simulink model "test_big_model"  (R2021b)
settings: Solver=ode23tb  StartTime=0.0  StopTime=ctrl_tm  MaxStep=0.01  RelTol=1e-3
values from neighbouring files (symbols this model uses):
  A = J    (= 0.066829)    [test_big.m]    (also in test_small.m = 0.000254045)
  B = b_m + b + (b/(N^2*n_g))    (= 0.00010739)    [test_big.m]    (also in test_small.m = 6e-07)
  ctrl_k = k    (= 0)    [controller_init.m]    (also in controller_init2.m = 1; controller_init3.m = 1)
  ctrl_max_vel = max_vel    (= 6)    [controller_init.m]    (also in controller_init2.m = 10; controller_init3.m = 8)
  ctrl_mp = mp    (= 3)    [controller_init.m]    (also in controller_init2.m; controller_init3.m)
  ctrl_t1 = (tm-k*tm)/2    (= 3.75)    [controller_init.m]    (also in controller_init2.m = 0; controller_init3.m = 0)
  ctrl_t3 = ctrl_t1    (= 3.75)    [controller_init.m]    (also in controller_init2.m = 0; controller_init3.m = 0)
  ctrl_tm = tm    (= 7.5)    [controller_init.m]    (also in controller_init2.m = 3; controller_init3.m = 20)
  D = (mu_s*cos(angl) + sin(angl)) * r_p*(m_l+m_b)*g/(N*n_g)    [test_big.m]    (also in test_small.m = 0.113379075)
  Ke = 0.0537    [test_big.m]    (also in test_small.m = 0.0168)
  L = 0.0308e-3    (= 3.08e-05)    [test_big.m]    (also in test_small.m = 0.000333)
  max_i = 10    [test_big.m]
  MP_ON = 1    [test_big.m]
  N = (1:0.1:50)    [gear_ratio_code_1.m]    (also in test_big.m = 1; test_small.m = 1)
  R = 0.0821    [test_big.m]    (also in test_small.m = 3.17)
  r_p = 0.5e-1    (= 0.05)    [test_big.m]    (also in test_small.m = 0.005)
  USE_MAX_OP = 0    [test_big.m]
  V = 24    [test_big.m]    (also in test_small.m = 12)
undefined symbols (not defined in the file or in its folder): sigbuilder_block
libraries: slpidlib x1, simulink x1, eePwmGenerator x1
settings Model: Creator=marcelafunyah  LastModifiedBy=marcelafunyah

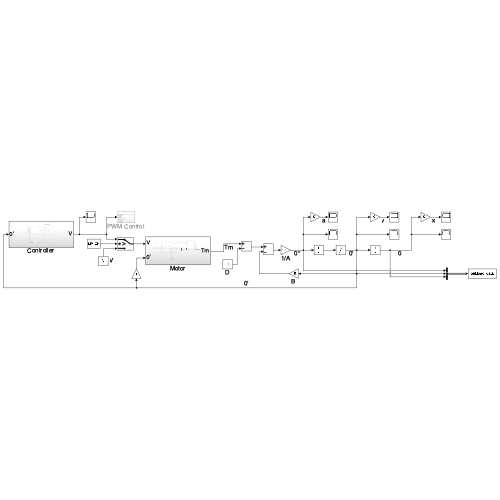
[thumbnail: Simulink's stored preview of the top-level diagram]
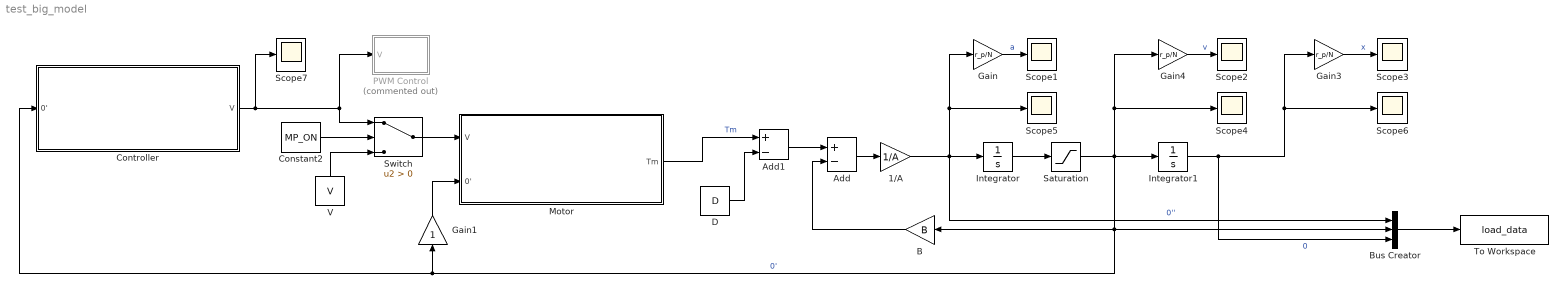
== system test_big_model ==
  1/A : Gain  Gain=1/A
  Add : Sum  Inputs=+-
  Add1 : Sum  Inputs=+-
  B : Gain  Gain=B
  Bus Creator : BusCreator  Inputs=3
  Constant2 : Constant  Value=MP_ON
  Controller : Subsystem
  D : Constant  Value=D
  Gain : Gain  Gain=r_p/N
  Gain1 : Gain
  Gain3 : Gain  Gain=r_p/N
  Gain4 : Gain  Gain=r_p/N
  Integrator : Integrator
  Integrator1 : Integrator
  Motor : Subsystem
  PWM Control : Subsystem  Commented=on
  Saturation : Saturate  UpperLimit=inf  LowerLimit=0
  Scope{1..7} (7 alike) : Scope
  Switch : Switch  Criteria=u2 > Threshold
  To Workspace : ToWorkspace  VariableName=load_data  SaveFormat=Timeseries  SampleTime=-1
  V : Constant  Value=V
  wires:
  Integrator/1 -> Saturation/1
  Integrator1/1 -> Bus Creator/3, Gain3/1, Scope6/1  "0"
  1/A/1 -> Bus Creator/1, Gain/1, Scope5/1, Integrator/1  "0''"
  B/1 -> Add/2
  Gain/1 -> Scope1/1  "a"
  Gain4/1 -> Scope2/1  "v"
  Gain3/1 -> Scope3/1  "x"
  Add/1 -> 1/A/1
  D/1 -> Add1/2
  Add1/1 -> Add/1
  Motor/1(Tm) -> Add1/1  "Tm"
  Controller/1(V) -> Scope7/1, PWM Control/1(V), Switch/1
  V/1 -> Switch/3
  Saturation/1 -> Gain4/1, Scope4/1, Controller/1(0'), Gain1/1, Bus Creator/2, B/1, Integrator1/1  "0'"
  Switch/1 -> Motor/1(V)
  Constant2/1 -> Switch/2
  Bus Creator/1 -> To Workspace/1
  Gain1/1 -> Motor/2(0')

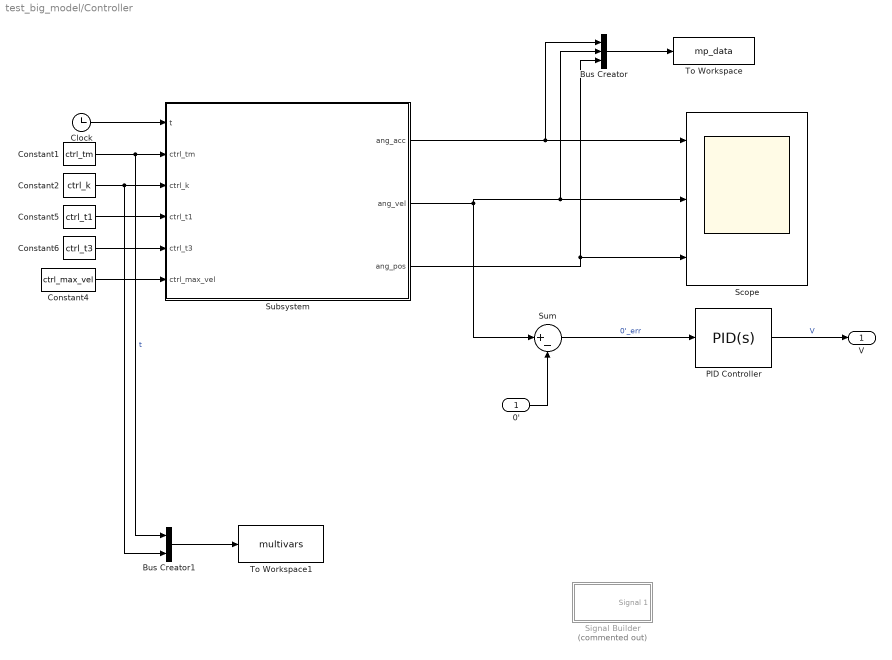
== system test_big_model/Controller ==
  0' : Inport
  Bus Creator : BusCreator  Inputs=3
  Bus Creator1 : BusCreator  Inputs=2
  Clock : Clock
  Constant1 : Constant  Value=ctrl_tm
  Constant2 : Constant  Value=ctrl_k
  Constant4 : Constant  Value=ctrl_max_vel
  Constant5 : Constant  Value=ctrl_t1
  Constant6 : Constant  Value=ctrl_t3
  PID Controller : slpidlib/PID Controller  Controller=PID  Form=Parallel  TimeDomain=Continuous-time  UseExternalTs=off  SampleTime=-1  IntegratorMethod=Forward Euler  FilterMethod=Forward Euler  ControllerParametersSource=internal  P=1452.99988960196  I=1492324.06717595  D=0.320852437052245  UseFilter=on  N=33719.8695903616  TunerSelectOption=Transfer Function Based (PID Tuner App)  InitialConditionSource=internal  InitialConditionForIntegrator=0  InitialConditionForFilter=0  DifferentiatorICPrevScaledInput=0  ExternalReset=none  TrackingMode=off  Kt=1  LimitOutput=on  SatLimitsSource=internal  UpperSaturationLimit=12  LowerSaturationLimit=0  LinearizeAsGain=on  AntiWindupMode=none  Kb=1  POutMin=[]  POutMax=[]  IOutMin=[]  IOutMax=[]  DOutMin=[]  DOutMax=[]  NOutMin=[]  NOutMax=[]  SumOutMin=[]  SumOutMax=[]  SaturationOutMin=[]  SaturationOutMax=[]  PParamMin=[]  PParamMax=[]  IParamMin=[]  IParamMax=[]  DParamMin=[]  DParamMax=[]  NParamMin=[]  NParamMax=[]  KbParamMin=[]  KbParamMax=[]  KtParamMin=[]  KtParamMax=[]  KbOutMin=[]  KbOutMax=[]  KtOutMin=[]  KtOutMax=[]  IntegratorOutMin=[]  IntegratorOutMax=[]  FilterOutMin=[]  FilterOutMax=[]  SumI1OutMin=[]  SumI1OutMax=[]  SumI2OutMin=[]  SumI2OutMax=[]  SumI3OutMin=[]  SumI3OutMax=[]  SumI4OutMin=[]  SumI4OutMax=[]  SumDOutMin=[]  SumDOutMax=[]  DifferentiatorOutMin=[]  DifferentiatorOutMax=[]  FilterDiffOutCoefMin=[]  FilterDiffOutCoefMax=[]  ReciprocalOutMin=[]  ReciprocalOutMax=[]  SumDenOutMin=[]  SumDenOutMax=[]  SumNumOutMin=[]  SumNumOutMax=[]  DivideOutMin=[]  DivideOutMax=[]  UdiffTsProdOutMin=[]  UdiffTsProdOutMax=[]  NTsProdOutMin=[]  NTsProdOutMax=[]  UintegralTsProdOutMin=[]  UintegralTsProdOutMax=[]  UngainTsProdOutMin=[]  UngainTsProdOutMax=[]  IntegratorContinuousStateAttributes=''  IntegratorStateMustResolveToSignalObject=off  IntegratorRTWStateStorageClass=Auto  FilterContinuousStateAttributes=''  FilterStateMustResolveToSignalObject=off  FilterRTWStateStorageClass=Auto  ParallelPVariant=InternalParameters  IdealPVariant=Disabled  IVariant=InternalParameters  DVariant=InternalParameters  IntegratorVariant=Continuous  SatVariant=Enabled  AWVariant=Passthrough  PCopyVariant=Disabled  TRVariant=Disabled  FdbkBlocksVariant=Forward  IdealPFdbkVariant=Disabled  SatFdbkVariant=Disabled  DerivativeFilterVariant=ContFilter  NVariant=InternalParameters  NCopyVariant=Disabled  FilterICVariant=InternalICsFilter  IntegratorICVariant=InternalICs  ExternalResetVariant=Disabled  TRSumVariant=Passthrough  SumFdbkVariant=Disabled  SumVariant=Sum_PID  TsampFilterVariant=InternalTs  TsampNgainVariant=Passthrough  TsampIntegralVariant=Passthrough  ExternalSaturationOutDataTypeStr=Inherit: Same as second input
  Scope : Scope  NumInputPorts=3
  Signal Builder : Subsystem  Tag=STV Subsys  Commented=on  LoadFcn=sigbuilder_block('load');  StartFcn=sigbuilder_block('start');  StopFcn=sigbuilder_block('stop');  ClipboardFcn=sigbuilder_block('clipboard');  mask(Sigbuilder block){tuvar=[0:10]}
      mask help: Simulink:masks:SigbuilderBlock_MD
      mask init:
      | if ~strcmp(get_param(bdroot(gcbh),'SimulationStatus'),'stopped') tuvar = sigbuilder_block('maskInit'); end
      settings: CopyFcn=sigbuilder_block('copy');  DeleteFcn=sigbuilder_block('delete');  ModelCloseFcn=sigbuilder_block('modelClose');  PreSaveFcn=sigbuilder_block('preSave');  PauseFcn=sigbuilder_block('pause');  ContinueFcn=sigbuilder_block('continue');  NameChangeFcn=sigbuilder_block('namechange');  OpenFcn=sigbuilder_block('open',[437.6 199.2 550.4 400 ]);  CloseFcn=sigbuilder_block('close');
      mask Display: plot(0, 0, 100, 100,[2, 2, 32, 32, 2], [68, 8, 8, 68, 68],[32, 2], [38, 38], [32, 19, 2],[53, 60, 44], [32, 17, 17, 2],[16, 16, 31, 31]);txt = getActiveGroup(gcbh);text(2, 100, txt,'verticalAlignment', 'top');
  Subsystem : Subsystem
  Sum : Sum  Inputs=|+-
  To Workspace : ToWorkspace  VariableName=mp_data  SaveFormat=Timeseries  SampleTime=-1
      settings: Save2DSignal=2-D array (concatenate along first dimension)
  To Workspace1 : ToWorkspace  VariableName=multivars  SaveFormat=Timeseries  SampleTime=-1
      settings: Save2DSignal=2-D array (concatenate along first dimension)
  V : Outport
  wires:
  Sum/1 -> PID Controller/1  "0'_err"
  PID Controller/1 -> V/1  "V"
  0'/1 -> Sum/2
  Bus Creator/1 -> To Workspace/1
  Subsystem/2(ang_vel) -> Bus Creator/2, Scope/2, Sum/1
  Subsystem/1(ang_acc) -> Bus Creator/1, Scope/1
  Subsystem/3(ang_pos) -> Bus Creator/3, Scope/3
  Clock/1 -> Subsystem/1(t)
  Constant1/1 -> Bus Creator1/1, Subsystem/2(ctrl_tm)  "t"
  Constant2/1 -> Bus Creator1/2, Subsystem/3(ctrl_k)
  Constant4/1 -> Subsystem/6(ctrl_max_vel)
  Bus Creator1/1 -> To Workspace1/1
  Constant6/1 -> Subsystem/5(ctrl_t3)
  Constant5/1 -> Subsystem/4(ctrl_t1)

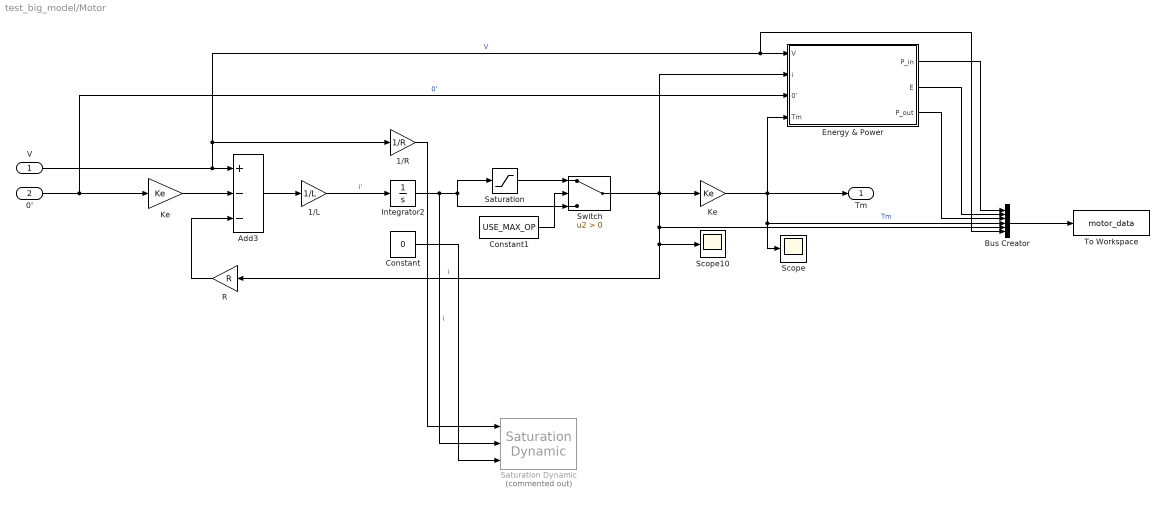
== system test_big_model/Motor ==
  V : Inport
  0' : Inport  Port=2
  1/L : Gain  Gain=1/L
  1/R : Gain  Gain=1/R
  Add3 : Sum  Inputs=+--
  Bus Creator : BusCreator  Inputs=6
  Constant : Constant  Value=0
  Constant1 : Constant  Value=USE_MAX_OP
  Energy & Power : Subsystem
  Integrator2 : Integrator
  Ke : Gain  Gain=Ke
  "Ke " : Gain  Gain=Ke
  R : Gain  Gain=R
  Saturation : Saturate  UpperLimit=max_i  LowerLimit=-inf
  Saturation Dynamic : simulink/Discontinuities/Saturation Dynamic  Commented=on  OutMin=[]  OutMax=[]  OutDataTypeStr=Inherit: Same as second input  OutDataType=fixdt(1, 16)  OutScaling=2^-10  DoSatur=off
  Scope : Scope
  Scope10 : Scope
  Switch : Switch  Criteria=u2 > Threshold
  To Workspace : ToWorkspace  VariableName=motor_data  SaveFormat=Timeseries  SampleTime=-1
  Tm : Outport
  wires:
  R/1 -> Add3/3
  Add3/1 -> 1/L/1
  "Ke "/1 -> Tm/1, Energy & Power/4(Tm), Scope/1, Bus Creator/4  "Tm"
  1/L/1 -> Integrator2/1  "i'"
  Ke/1 -> Add3/2
  V/1 -> Bus Creator/6, Energy & Power/1(V), 1/R/1, Add3/1  "V"
  0'/1 -> Ke/1, Energy & Power/3(0')  "0'"
  Integrator2/1 -> Switch/3, Saturation/1, Saturation Dynamic/2  "i"
  1/R/1 -> Saturation Dynamic/1
  Constant/1 -> Saturation Dynamic/3
  Bus Creator/1 -> To Workspace/1
  Energy & Power/3(P_out) -> Bus Creator/3
  Energy & Power/2(E) -> Bus Creator/2
  Energy & Power/1(P_in) -> Bus Creator/1
  Switch/1 -> Energy & Power/2(i), R/1, Scope10/1, Bus Creator/5, "Ke "/1  "i"
  Saturation/1 -> Switch/1
  Constant1/1 -> Switch/2

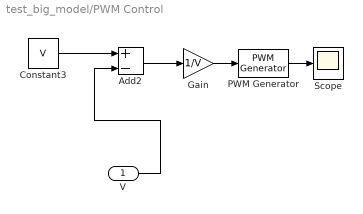
== system test_big_model/PWM Control ==
  V : Inport
  Add2 : Sum  Inputs=+-
  Constant3 : Constant  Value=V
  Gain : Gain  Gain=1/V
  PWM Generator : eePwmGenerator/PWM Generator  CarrCount=Up  Tper=0.001  Tdelay=0  Ts=0
  Scope : Scope
  wires:
  PWM Generator/1 -> Scope/1
  Gain/1 -> PWM Generator/1
  Constant3/1 -> Add2/1
  V/1 -> Add2/2
  Add2/1 -> Gain/1

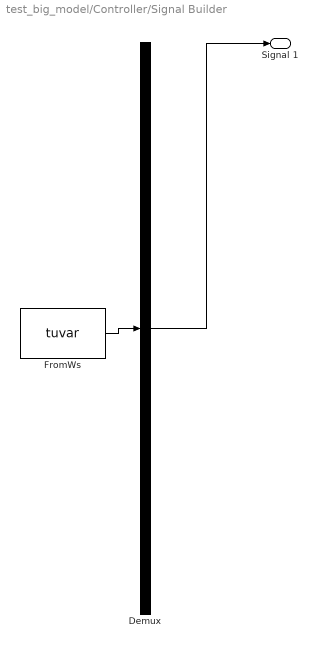
== system test_big_model/Controller/Signal Builder ==
  Demux : Demux  Tag=STV Demux  Outputs=1
      settings: DisplayOption=none
  FromWs : FromWorkspace  Tag=STV FromWs  VariableName=tuvar
      SigBuilderData=|
      | common.afterFinalStr = 'Extrapolate'
      | common.sampleTime = 0
      | dataSet.timeRange = [0 5]
      | dataSet.name = 'Group 1'
      | sbobj.Groups.Name = 'Group 1'
      | sbobj.Groups.Signals.Name = 'Signal 1'
      | sbobj.Groups.Signals.XData = [0 5]
      | sbobj.Groups.Signals.YData = [0.75 0.75]
      | sbobj.Groups.TimeRange = [0 5]
  Signal 1 : Outport  Tag=STV Outport
  wires:
  Demux/1 -> Signal 1/1
  FromWs/1 -> Demux/1

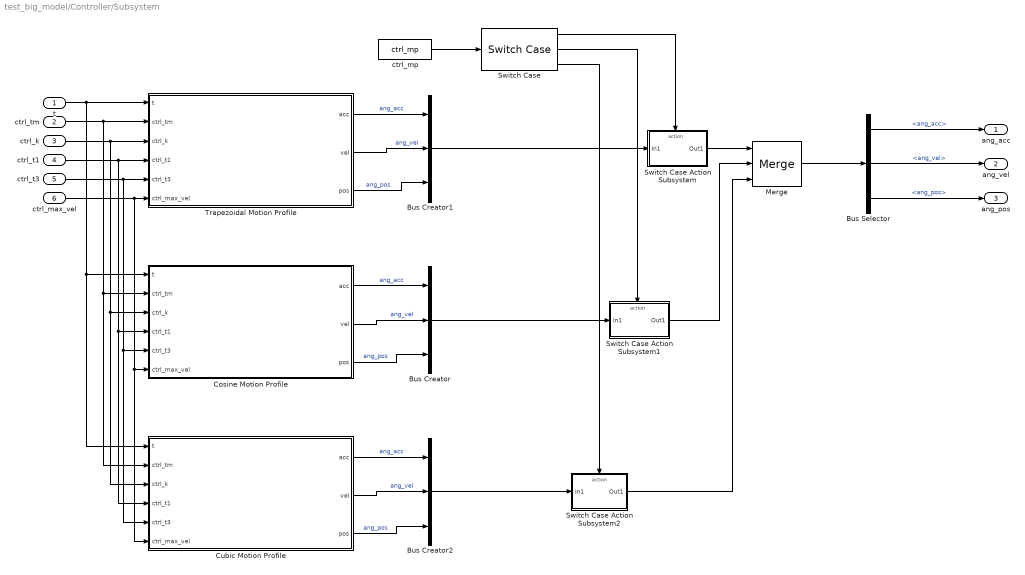
== system test_big_model/Controller/Subsystem ==
  t : Inport
  ctrl_tm : Inport  Port=2
  ctrl_k : Inport  Port=3
  ctrl_t1 : Inport  Port=4
  ctrl_t3 : Inport  Port=5
  ctrl_max_vel : Inport  Port=6
  Bus Creator : BusCreator  Inputs=3
  Bus Creator1 : BusCreator  Inputs=3
  Bus Creator2 : BusCreator  Inputs=3
  Bus Selector : BusSelector  OutputSignals=ang_acc,ang_vel,ang_pos
  Cosine Motion Profile : MATLAB Function  TreatAsAtomicUnit=on
  Cubic Motion Profile : MATLAB Function  TreatAsAtomicUnit=on
  Merge : Merge  Inputs=3
  Switch Case : SwitchCase  CaseConditions={1,2,3}  ShowDefaultCase=off
  Switch Case Action Subsystem : Subsystem  TreatAsAtomicUnit=on
  Switch Case Action Subsystem1 : Subsystem  TreatAsAtomicUnit=on
  Switch Case Action Subsystem2 : Subsystem  TreatAsAtomicUnit=on
  Trapezoidal Motion Profile : MATLAB Function  TreatAsAtomicUnit=on
  ctrl_mp : Constant  Value=ctrl_mp
  ang_acc : Outport
  ang_vel : Outport  Port=2
  ang_pos : Outport  Port=3
  wires:
  Cosine Motion Profile/1(acc) -> Bus Creator/1  "ang_acc"
  Cosine Motion Profile/3(pos) -> Bus Creator/3  "ang_pos"
  Cosine Motion Profile/2(vel) -> Bus Creator/2  "ang_vel"
  Switch Case/1 -> Switch Case Action Subsystem/Action
  Trapezoidal Motion Profile/1(acc) -> Bus Creator1/1  "ang_acc"
  Trapezoidal Motion Profile/2(vel) -> Bus Creator1/2  "ang_vel"
  Trapezoidal Motion Profile/3(pos) -> Bus Creator1/3  "ang_pos"
  Bus Creator1/1 -> Switch Case Action Subsystem/1(In1)
  Switch Case Action Subsystem/1(Out1) -> Merge/1
  Switch Case/2 -> Switch Case Action Subsystem1/Action
  Bus Creator/1 -> Switch Case Action Subsystem1/1(In1)
  Switch Case Action Subsystem1/1(Out1) -> Merge/2
  Merge/1 -> Bus Selector/1
  Bus Selector/1 -> ang_acc/1  "<ang_acc>"
  Bus Selector/2 -> ang_vel/1  "<ang_vel>"
  Bus Selector/3 -> ang_pos/1  "<ang_pos>"
  ctrl_mp/1 -> Switch Case/1
  Cubic Motion Profile/1(acc) -> Bus Creator2/1  "ang_acc"
  t/1 -> Cubic Motion Profile/1(t), Cosine Motion Profile/1(t), Trapezoidal Motion Profile/1(t)
  ctrl_max_vel/1 -> Cubic Motion Profile/6(ctrl_max_vel), Cosine Motion Profile/6(ctrl_max_vel), Trapezoidal Motion Profile/6(ctrl_max_vel)
  ctrl_tm/1 -> Cubic Motion Profile/2(ctrl_tm), Cosine Motion Profile/2(ctrl_tm), Trapezoidal Motion Profile/2(ctrl_tm)
  Cubic Motion Profile/2(vel) -> Bus Creator2/2  "ang_vel"
  ctrl_k/1 -> Cubic Motion Profile/3(ctrl_k), Cosine Motion Profile/3(ctrl_k), Trapezoidal Motion Profile/3(ctrl_k)
  Bus Creator2/1 -> Switch Case Action Subsystem2/1(In1)
  Cubic Motion Profile/3(pos) -> Bus Creator2/3  "ang_pos"
  Switch Case/3 -> Switch Case Action Subsystem2/Action
  Switch Case Action Subsystem2/1(Out1) -> Merge/3
  ctrl_t1/1 -> Cubic Motion Profile/4(ctrl_t1), Cosine Motion Profile/4(ctrl_t1), Trapezoidal Motion Profile/4(ctrl_t1)
  ctrl_t3/1 -> Cubic Motion Profile/5(ctrl_t3), Cosine Motion Profile/5(ctrl_t3), Trapezoidal Motion Profile/5(ctrl_t3)

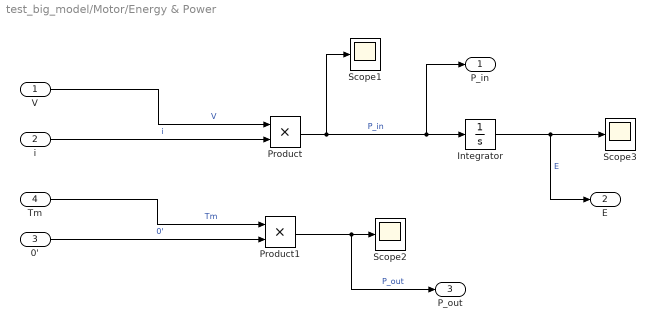
== system test_big_model/Motor/Energy & Power ==
  V : Inport
  i : Inport  Port=2
  0' : Inport  Port=3
  Tm : Inport  Port=4
  Integrator : Integrator
  Product : Product
  Product1 : Product
  Scope1 : Scope
  Scope2 : Scope
  Scope3 : Scope
  P_in : Outport
  E : Outport  Port=2
  P_out : Outport  Port=3
  wires:
  V/1 -> Product/1  "V"
  i/1 -> Product/2  "i"
  Product/1 -> P_in/1, Integrator/1, Scope1/1  "P_in"
  Integrator/1 -> E/1, Scope3/1  "E"
  Tm/1 -> Product1/1  "Tm"
  0'/1 -> Product1/2  "0'"
  Product1/1 -> P_out/1, Scope2/1  "P_out"

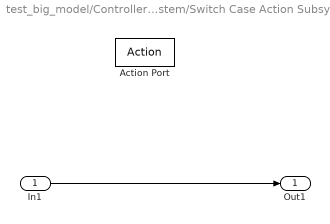
== system test_big_model/Controller/Subsystem/Switch Case Action Subsystem ==
  In1 : Inport
  Action Port : ActionPort  ActionPortLabel=case [ 1 ]:
  Out1 : Outport
  wires:
  In1/1 -> Out1/1

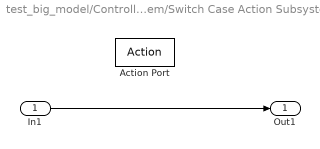
== system test_big_model/Controller/Subsystem/Switch Case Action Subsystem1 ==
  In1 : Inport
  Action Port : ActionPort  ActionPortLabel=case [ 2 ]:
  Out1 : Outport
  wires:
  In1/1 -> Out1/1

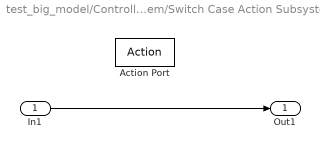
== system test_big_model/Controller/Subsystem/Switch Case Action Subsystem2 ==
  In1 : Inport
  Action Port : ActionPort  ActionPortLabel=case [ 3 ]:
  Out1 : Outport
  wires:
  In1/1 -> Out1/1

== matlab function test_big_model/Controller/Subsystem/Cosine Motion Profile ==
  data: t input; acc output; vel output; pos output; ctrl_tm input; ctrl_k input; ctrl_t1 input; ctrl_t3 input; ctrl_max_vel input
function [acc,vel,pos] = fcn(t, ctrl_tm, ctrl_k, ctrl_t1, ctrl_t3, ctrl_max_vel)

tm = ctrl_tm;
k = ctrl_k;

t1 = ctrl_t1;
t3 = ctrl_t3;

max_ang_vel = ctrl_max_vel;


% ta = 0;
% tb = ta + 0.5 * (tm - k*tm);
% tc = tb + k*tm;
% td = tm;
% 
% t_acc = tb - ta;
% t_dec = td - tc;


ta = 0;
tb = ta + t1;
tc = tb + k*tm;
td = tm;

t_acc = t1;
t_dec = t3;

thet1 = pi/t_acc;
thet3 = pi/t_dec;


if (t>=ta) && (t<=tb)
    ang_acc = max_ang_vel*(thet1*sin(thet1*t))/2;
    ang_vel = max_ang_vel*(1-cos(thet1*t))/2;
    ang_pos = max_ang_vel*(t-sin(thet1*t)/thet1)/2;

elseif (t>tb) && (t<=tc)
    ang_acc = 0;
    ang_vel = max_ang_vel;
    ang_pos = max_ang_vel*(t-t_acc/2);

elseif (t>tc) && (t<=td)
    tprm = t - tm + t_dec;
    ang_acc = -max_ang_vel*(thet3*sin(thet3*tprm))/2;
    ang_vel = max_ang_vel*(1+cos(thet3*tprm))/2;
    ang_pos = max_ang_vel*(tm - t_acc/2 - t_dec) + max_ang_vel*(tprm+sin(thet3*tprm)/thet3)/2;
else
    tprm = tm - tm + t_dec;
    ang_acc = 0;
    ang_vel = 0;
    ang_pos = max_ang_vel*(tm - t_acc/2 - t_dec) + max_ang_vel*(tprm+sin(thet3*tprm)/thet3)/2;
end



acc = ang_acc;
vel = ang_vel;
pos = ang_pos;

== matlab function test_big_model/Controller/Subsystem/Trapezoidal Motion Profile ==
  data: t input; acc output; vel output; pos output; ctrl_tm input; ctrl_k input; ctrl_t1 input; ctrl_t3 input; ctrl_max_vel input
function [acc,vel,pos] = fcn(t, ctrl_tm, ctrl_k, ctrl_t1, ctrl_t3, ctrl_max_vel)

    tm = ctrl_tm;
    k = ctrl_k;

    t1 = ctrl_t1;
    t3 = ctrl_t3;

    vel = ctrl_max_vel;

    ta = 0;
    tb = ta + t1;
    tc = tb + k*tm;
    td = tm;

    A1 =vel / t1;
    A2 =vel / t3;


    if (t>=ta) && (t<=tb)
        ang_acc = A1;
        ang_vel = A1 * t;
        ang_pos = 0.5 * A1 * t^2; 
    elseif (t>tb) && (t<=tc)
        ang_acc = 0;
        ang_vel = A1 * tb;
        ang_pos = (0.5 * A1 * tb^2) + (A1 * tb) * (t - tb); 
    elseif (t>tc) && (t<=td)
        ang_acc = -A2;
        ang_vel = (A1 * tb) - A2*(t-tc);
        ang_pos = (0.5 * A1 * tb^2) + (A1 * tb) * (tc - tb) + (A1 * tb) * (t - tc) + (A2 * tc) * (t - tc) - 0.5 * A2 * (t^2 - tc^2);
    else
        ang_acc = 0;
        ang_vel = 0;
        ang_pos = (0.5 * A1 * tb^2) + (A1 * tb) * (tc - tb) + (A1 * tb) * (tm - tc) + (A2 * tc) * (tm - tc) - 0.5 * A2 * (tm^2 - tc^2);
    end


acc = ang_acc;
vel = ang_vel;
pos = ang_pos;

== matlab function test_big_model/Controller/Subsystem/Cubic Motion Profile ==
  data: t input; acc output; vel output; pos output; ctrl_tm input; ctrl_k input; ctrl_t1 input; ctrl_t3 input; ctrl_max_vel input
function [acc,vel,pos] = fcn(t, ctrl_tm, ctrl_k, ctrl_t1, ctrl_t3, ctrl_max_vel)

tm = ctrl_tm;
k = ctrl_k;

t1 = ctrl_t1;
t3 = ctrl_t3;

max_ang_vel = ctrl_max_vel;

% ta = 0;
% tb = ta + 0.5 * (tm - k*tm);
% tc = tb + k*tm;
% td = tm;
% 
% t_acc = tb - ta;
% t_dec = td - tc;

ta = 0;
tb = ta + t1;
tc = tb + k*tm;
td = tm;

t_acc = t1;
t_dec = t3;


if (t>=ta) && (t<=tb)
    ang_acc = 2*max_ang_vel/t_acc - 2*max_ang_vel*t/t_acc^2;
    ang_vel = 2*max_ang_vel*t/t_acc - max_ang_vel*t^2/t_acc^2;
    ang_pos = max_ang_vel*t^2/t_acc- max_ang_vel*t^3/(3*t_acc^2);
elseif (t>tb) && (t<=tc)
    ang_acc = 0;
    ang_vel = max_ang_vel;
    ang_pos = max_ang_vel*tb^2/t_acc - max_ang_vel*tb^3/(3*t_acc^2) + max_ang_vel*(t-tb);
elseif (t>tc) && (t<=td)
    ang_acc = -2*max_ang_vel*(t-tc)/t_dec^2;
    ang_vel = max_ang_vel - max_ang_vel*(t-tc)^2/t_dec^2;
    ang_pos = max_ang_vel*tb^2/t_acc - max_ang_vel*tb^3/(3*t_acc^2) + max_ang_vel*(tc-tb) + max_ang_vel*(t-tc) - max_ang_vel*(t-tc)^3/(3*t_dec^2);
else
    ang_acc = 0;
    ang_vel = 0;
    ang_pos = max_ang_vel*tb^2/t_acc - max_ang_vel*tb^3/(3*t_acc^2) + max_ang_vel*(tc-tb) + max_ang_vel*(tm-tc) - max_ang_vel*(tm-tc)^3/(3*t_dec^2);
end



acc = ang_acc;
vel = ang_vel;
pos = ang_pos;
